simulink subsystem "EX"  (R2024b)
settings: Solver=VariableStepAuto  StartTime=0.0  StopTime=10.0  RelTol=1e-3
settings Model: Creator=stefano  LastModifiedBy=stefano

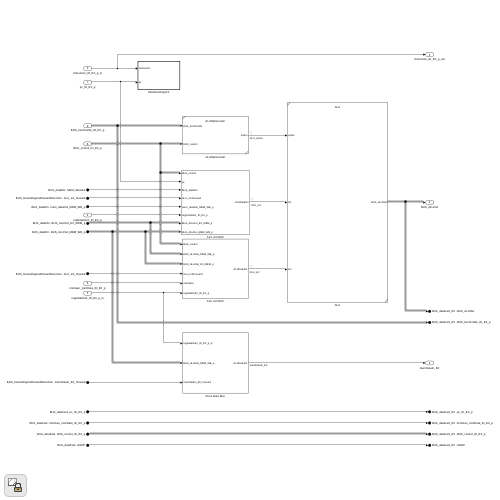
[thumbnail: Simulink's stored preview of the top-level diagram]
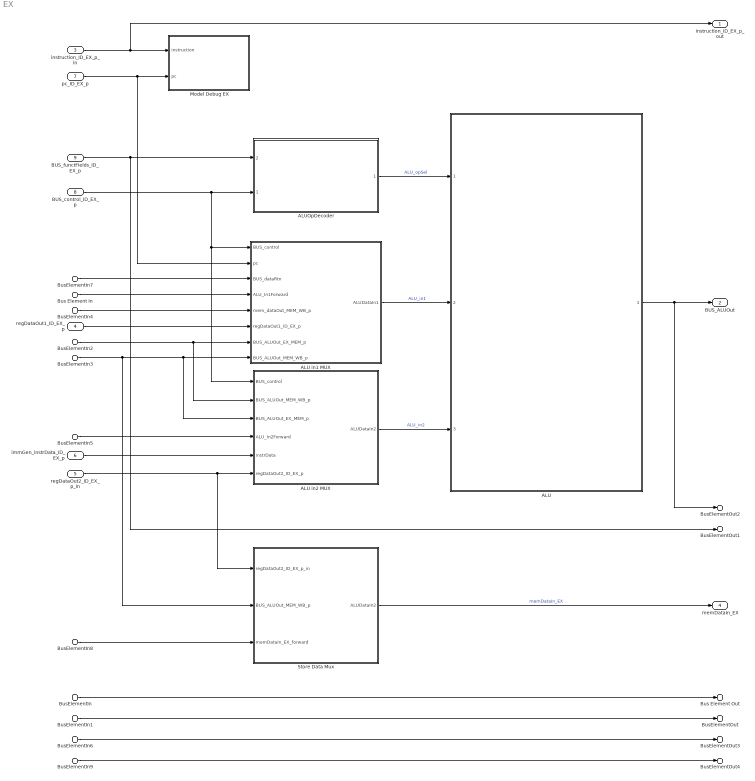
== system EX ==
  BusElementIn4 : Inport  PortName=BUS_dataRtn  Element=mem_dataOut_MEM_WB_p
  BusElementIn2 : Inport  PortName=BUS_dataRtn  Element=BUS_ALUOut_EX_MEM_p
  BusElementIn3 : Inport  PortName=BUS_dataRtn  Element=BUS_ALUOut_MEM_WB_p
  BusElementIn7 : Inport  PortName=BUS_dataRtn  Element=MEM_dataOut
  BusElementIn5 : Inport  Port=2  PortName=BUS_forwardingAndHazardDetection  Element=ALU_in2_forward
  Bus Element In : Inport  Port=2  PortName=BUS_forwardingAndHazardDetection  Element=ALU_in1_forward
  BusElementIn8 : Inport  Port=2  PortName=BUS_forwardingAndHazardDetection  Element=memDataIn_EX_forward
  instruction_ID_EX_p_in : Inport  Port=3
  regDataOut1_ID_EX_p : Inport  Port=4
  regDataOut2_ID_EX_p_in : Inport  Port=5
  immGen_instrData_ID_EX_p : Inport  Port=6
  pc_ID_EX_p : Inport  Port=7
  BUS_control_ID_EX_p : Inport  Port=8
  BUS_functFields_ID_EX_p : Inport  Port=9
  BusElementIn : Inport  Port=10  PortName=BUS_dataFwd  Element=pc_ID_EX_p
  BusElementIn1 : Inport  Port=10  PortName=BUS_dataFwd  Element=immGen_instrData_ID_EX_p
  BusElementIn6 : Inport  Port=10  PortName=BUS_dataFwd  Element=BUS_control_ID_EX_p
  BusElementIn9 : Inport  Port=10  PortName=BUS_dataFwd  Element=retireInstruction
  ALU : Subsystem  ReferencedSubsystem=ALU
  ALU in1 MUX : Subsystem
  ALU in2 MUX : Subsystem
  ALUOpDecoder : Subsystem  ReferencedSubsystem=ALUOpDecoder
      settings: PortSchema="{\"entries\":[{\"content\":{\"sides\":[{\"content\":{\"connectorIds\":[\"In2\",\"In1\"]},\"type\":\"ConnectorPlacement.EquallySpacedRectSide\",\"uuid\":\"84e38179-b753-4f9f-98d7-a5402cb96b34\"},{\"content\":{\"connectorIds\":[\"Out1\"],\"side\":\"RIGHT\"},\"type\":\"ConnectorPlacement.EquallySpacedRectSide\",\"uuid\":\"5e360d21-5990-472e-9592-0fd1cc8b696e\"},{\"content\":{\"side\":\"TOP\"},\"type\":\"ConnectorPlacement.EquallySpacedRectSide\",\"uuid\":\"5c8518ac-bbb7-4afc-993e-2131e568568f\"}]},\"type\":\"ConnectorPlacement.EquallySpacedConnector\",\"uuid\":\"ff1cba65-9491-4c35-afc2-2a91c7806151\"}],\"packageUris\":[\"http://schema.mathworks.com/mf0/Connector/R2020b\"],\"version\":\"1.0\"}"
  Model Debug EX : Subsystem  TreatAsAtomicUnit=on
  Store Data Mux : Subsystem
  instruction_ID_EX_p_out : Outport
  BUS_ALUOut : Outport  Port=2
  Bus Element Out : Outport  Port=3  PortName=BUS_dataFwd_EX  Element=pc_ID_EX_p
  BusElementOut : Outport  Port=3  PortName=BUS_dataFwd_EX  Element=immGen_instrData_ID_EX_p
  BusElementOut1 : Outport  Port=3  PortName=BUS_dataFwd_EX  Element=BUS_functFields_ID_EX_p
  BusElementOut2 : Outport  Port=3  PortName=BUS_dataFwd_EX  Element=BUS_ALUOut
  BusElementOut3 : Outport  Port=3  PortName=BUS_dataFwd_EX  Element=BUS_control_ID_EX_p
  BusElementOut4 : Outport  Port=3  PortName=BUS_dataFwd_EX  Element=retireInstruction
  memDataIn_EX : Outport  Port=4
  wires:
  instruction_ID_EX_p_in/1 -> Model Debug EX/1(instruction), instruction_ID_EX_p_out/1
  regDataOut1_ID_EX_p/1 -> ALU in1 MUX/6(regDataOut1_ID_EX_p)
  BusElementIn3/1 -> ALU in1 MUX/8(BUS_ALUOut_MEM_WB_p), ALU in2 MUX/3(BUS_ALUOut_EX_MEM_p), Store Data Mux/2(BUS_ALUOut_MEM_WB_p)
  BUS_functFields_ID_EX_p/1 -> ALUOpDecoder/2, BusElementOut1/1
  ALU in1 MUX/1(ALUDataIn1) -> ALU/2  "ALU_in1"
  ALU in2 MUX/1(ALUDataIn2) -> ALU/3  "ALU_in2"
  ALUOpDecoder/1 -> ALU/1  "ALU_opSel"
  BusElementIn2/1 -> ALU in1 MUX/7(BUS_ALUOut_EX_MEM_p), ALU in2 MUX/2(BUS_ALUOut_MEM_WB_p)
  BUS_control_ID_EX_p/1 -> ALUOpDecoder/1, ALU in1 MUX/1(BUS_control), ALU in2 MUX/1(BUS_control)
  immGen_instrData_ID_EX_p/1 -> ALU in2 MUX/5(instrData)
  pc_ID_EX_p/1 -> Model Debug EX/2(pc), ALU in1 MUX/2(pc)
  BusElementIn5/1 -> ALU in2 MUX/4(ALU_In2Forward)
  regDataOut2_ID_EX_p_in/1 -> ALU in2 MUX/6(regDataOut2_ID_EX_p), Store Data Mux/1(regDataOut2_ID_EX_p_in)
  BusElementIn4/1 -> ALU in1 MUX/5(mem_dataOut_MEM_WB_p)
  ALU/1 -> BUS_ALUOut/1, BusElementOut2/1
  Bus Element In/1 -> ALU in1 MUX/4(ALU_In1Forward)
  BusElementIn/1 -> Bus Element Out/1
  BusElementIn1/1 -> BusElementOut/1
  BusElementIn6/1 -> BusElementOut3/1
  BusElementIn7/1 -> ALU in1 MUX/3(BUS_dataRtn)
  Store Data Mux/1(ALUDataIn2) -> memDataIn_EX/1  "memDataIn_EX"
  BusElementIn8/1 -> Store Data Mux/3(memDataIn_EX_forward)
  BusElementIn9/1 -> BusElementOut4/1

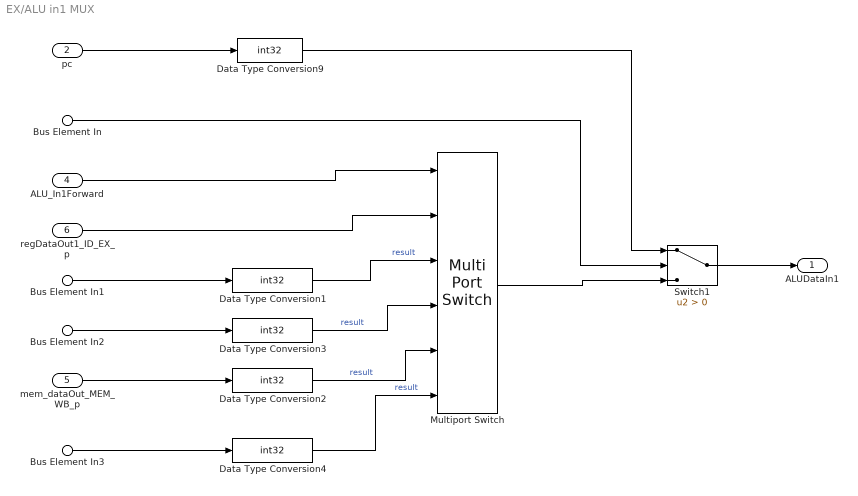
== system EX/ALU in1 MUX ==
  Bus Element In : Inport  PortName=BUS_control  Element=pcToALU
  pc : Inport  Port=2
  Bus Element In3 : Inport  Port=3  PortName=BUS_dataRtn
  ALU_In1Forward : Inport  Port=4
  mem_dataOut_MEM_WB_p : Inport  Port=5
  regDataOut1_ID_EX_p : Inport  Port=6
  Bus Element In2 : Inport  Port=7  PortName=BUS_ALUOut_EX_MEM_p  Element=result
  Bus Element In1 : Inport  Port=8  PortName=BUS_ALUOut_MEM_WB_p  Element=result
  Data Type Conversion{1..4} (4 alike) : DataTypeConversion  OutDataTypeStr=int32  ConvertRealWorld=Stored Integer (SI)  SaturateOnIntegerOverflow=off  RndMeth=Floor
  Data Type Conversion9 : DataTypeConversion  OutDataTypeStr=int32  SaturateOnIntegerOverflow=off  RndMeth=Floor
  Multiport Switch : MultiPortSwitch  DataPortOrder=Zero-based contiguous  Inputs=5  zeroidx=on  SaturateOnIntegerOverflow=off  InputSameDT=off
  Switch1 : Switch  Criteria=u2 > Threshold  SaturateOnIntegerOverflow=off  InputSameDT=off
  ALUDataIn1 : Outport
  wires:
  Data Type Conversion4/1 -> Multiport Switch/6  "result"
  Bus Element In3/1 -> Data Type Conversion4/1
  Bus Element In2/1 -> Data Type Conversion3/1
  Bus Element In1/1 -> Data Type Conversion1/1
  Data Type Conversion2/1 -> Multiport Switch/5  "result"
  mem_dataOut_MEM_WB_p/1 -> Data Type Conversion2/1
  Data Type Conversion1/1 -> Multiport Switch/3  "result"
  Data Type Conversion3/1 -> Multiport Switch/4  "result"
  Switch1/1 -> ALUDataIn1/1
  ALU_In1Forward/1 -> Multiport Switch/1
  Multiport Switch/1 -> Switch1/3
  Data Type Conversion9/1 -> Switch1/1
  Bus Element In/1 -> Switch1/2
  regDataOut1_ID_EX_p/1 -> Multiport Switch/2
  pc/1 -> Data Type Conversion9/1

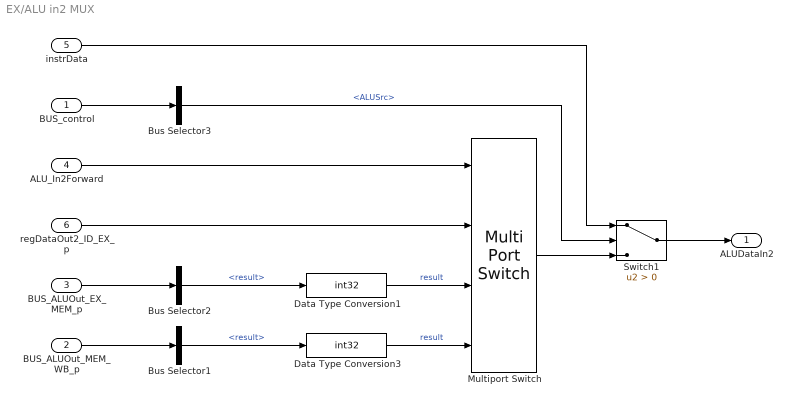
== system EX/ALU in2 MUX ==
  BUS_control : Inport
  BUS_ALUOut_MEM_WB_p : Inport  Port=2
  BUS_ALUOut_EX_MEM_p : Inport  Port=3
  ALU_In2Forward : Inport  Port=4
  instrData : Inport  Port=5
  regDataOut2_ID_EX_p : Inport  Port=6
  Bus Selector1 : BusSelector  OutputSignals=result
  Bus Selector2 : BusSelector  OutputSignals=result
  Bus Selector3 : BusSelector  OutputSignals=ALUSrc
  Data Type Conversion1 : DataTypeConversion  OutDataTypeStr=int32  ConvertRealWorld=Stored Integer (SI)  SaturateOnIntegerOverflow=off  RndMeth=Floor
  Data Type Conversion3 : DataTypeConversion  OutDataTypeStr=int32  ConvertRealWorld=Stored Integer (SI)  SaturateOnIntegerOverflow=off  RndMeth=Floor
  Multiport Switch : MultiPortSwitch  DataPortOrder=Zero-based contiguous  zeroidx=on  SaturateOnIntegerOverflow=off  InputSameDT=off
  Switch1 : Switch  Criteria=u2 > Threshold  SaturateOnIntegerOverflow=off  InputSameDT=off
  ALUDataIn2 : Outport
  wires:
  Multiport Switch/1 -> Switch1/3
  Bus Selector2/1 -> Data Type Conversion1/1  "<result>"
  Data Type Conversion1/1 -> Multiport Switch/3  "result"
  Data Type Conversion3/1 -> Multiport Switch/4  "result"
  ALU_In2Forward/1 -> Multiport Switch/1
  BUS_ALUOut_EX_MEM_p/1 -> Bus Selector2/1
  Switch1/1 -> ALUDataIn2/1
  Bus Selector1/1 -> Data Type Conversion3/1  "<result>"
  BUS_ALUOut_MEM_WB_p/1 -> Bus Selector1/1
  Bus Selector3/1 -> Switch1/2  "<ALUSrc>"
  regDataOut2_ID_EX_p/1 -> Multiport Switch/2
  BUS_control/1 -> Bus Selector3/1
  instrData/1 -> Switch1/1

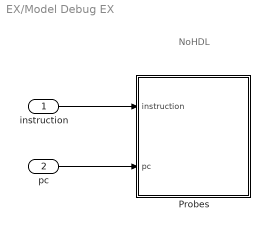
== system EX/Model Debug EX ==
  note: NoHDL
  instruction : Inport
  pc : Inport  Port=2
  Probes : Subsystem
  wires:
  pc/1 -> Probes/2(pc)
  instruction/1 -> Probes/1(instruction)

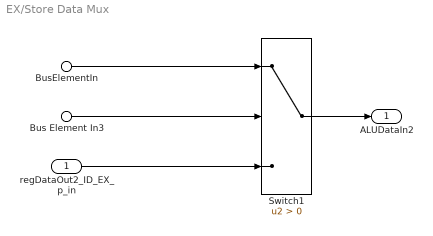
== system EX/Store Data Mux ==
  regDataOut2_ID_EX_p_in : Inport
  BusElementIn : Inport  Port=2  PortName=BUS_ALUOut_MEM_WB_p  Element=result
  Bus Element In3 : Inport  Port=3  PortName=memDataIn_EX_forward
  Switch1 : Switch  Criteria=u2 > Threshold  SaturateOnIntegerOverflow=off  InputSameDT=off
  ALUDataIn2 : Outport
  wires:
  Bus Element In3/1 -> Switch1/2
  BusElementIn/1 -> Switch1/1
  regDataOut2_ID_EX_p_in/1 -> Switch1/3
  Switch1/1 -> ALUDataIn2/1

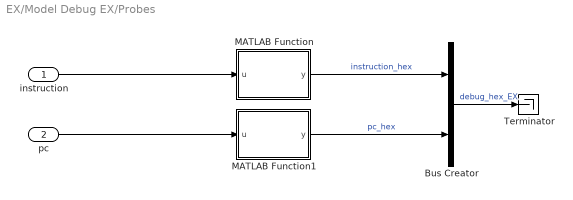
== system EX/Model Debug EX/Probes ==
  instruction : Inport
  pc : Inport  Port=2
  Bus Creator : BusCreator  Inputs=2
  MATLAB Function : MATLAB Function  TreatAsAtomicUnit=on
  MATLAB Function1 : MATLAB Function  TreatAsAtomicUnit=on
  Terminator : Terminator
  wires:
  MATLAB Function1/1(y) -> Bus Creator/2  "pc_hex"
  Bus Creator/1 -> Terminator/1  "debug_hex_EX"
  instruction/1 -> MATLAB Function/1(u)
  pc/1 -> MATLAB Function1/1(u)
  MATLAB Function/1(y) -> Bus Creator/1  "instruction_hex"

== matlab function EX/Model Debug EX/Probes/MATLAB Function1 ==
  data: u input; y output string
function y = toHex(u)

y = string(dec2hex(u, 8));

== matlab function EX/Model Debug EX/Probes/MATLAB Function ==
  data: u input; y output string
function y = toHex(u)

y = string(dec2hex(u, 8));
